simulink model "Model_Pendulum_14b"  (R2014b)
settings: Solver=ode45  StartTime=0.0  StopTime=10.0  RelTol=1e-3
undefined symbols (not defined in the file or in its folder): in
settings Model: Creator=Arek  LastModifiedBy=Arek
settings SolverCC: ZeroCrossAlgorithm=Adaptive

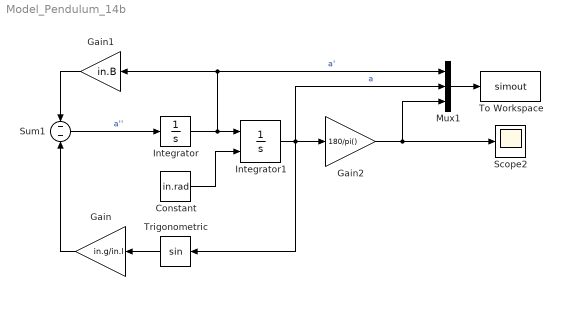
== system Model_Pendulum_14b ==
  Constant : Constant  Value=in.rad
  Gain : Gain  Gain=in.g/in.l
  Gain1 : Gain  Gain=in.B
  Gain2 : Gain  Gain=180/pi()
  Integrator : Integrator
  Integrator1 : Integrator  InitialConditionSource=external
  Mux1 : Mux  Inputs=3
  Scope2 : Scope
      settings: YMin=-10  YMax=10
  Sum1 : Sum  Inputs=-|-
  To Workspace : ToWorkspace  VariableName=simout  SaveFormat=Timeseries  SampleTime=-1
  Trigonometric : Trigonometry
  wires:
  Integrator/1 -> Mux1/1, Gain1/1, Integrator1/1  "a'"
  Constant/1 -> Integrator1/2
  Trigonometric/1 -> Gain/1
  Sum1/1 -> Integrator/1  "a''"
  Integrator1/1 -> Mux1/2, Trigonometric/1, Gain2/1  "a"
  Gain/1 -> Sum1/2
  Gain1/1 -> Sum1/1
  Gain2/1 -> Mux1/3, Scope2/1
  Mux1/1 -> To Workspace/1
